simulink model "Stateflow_calculator"  (R2016a)
settings: Solver=FixedStepDiscrete  StartTime=0.0  StopTime=10.0  RelTol=1e-3
settings Model: Creator=Mohamed Fawzy  LastModifiedBy=Mohamed Fawzy
settings OptimizationCC: DefaultParameterBehavior=Inlined  OptimizeModelRefInitCode=on  LifeSpan=1
settings RTWCC: SystemTargetFile=ert.tlc  GenCodeOnly=on  GenerateMakefile=off  TemplateMakefile=ert_default_tmf  GenerateReport=on  IncludeHyperlinkInReport=on  LaunchReport=on  GenerateTraceInfo=on  GenerateTraceReport=on  GenerateTraceReportSl=on  GenerateTraceReportSf=on  GenerateTraceReportEml=on
settings CodeAppCC: ForceParamTrailComments=on  IgnoreCustomStorageClasses=off  OperatorAnnotations=on  SimulinkDataObjDesc=on  SFDataObjDesc=on  MATLABFcnDesc=on  InsertBlockDesc=on  MATLABSourceComments=on
settings ERTTargetCC: GenerateSampleERTMain=on  SuppressErrorStatus=on  InlinedParameterPlacement=NonHierarchical  ERTCustomFileTemplate=example_file_process.tlc

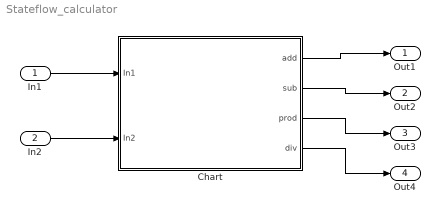
== system Stateflow_calculator ==
  In1 : Inport  OutDataTypeStr=uint8
  In2 : Inport  Port=2  OutDataTypeStr=uint8
  Chart : Stateflow chart  TreatAsAtomicUnit=on
  Out1 : Outport  OutDataTypeStr=uint8
  Out2 : Outport  Port=2  OutDataTypeStr=uint8
  Out3 : Outport  Port=3  OutDataTypeStr=uint16
  Out4 : Outport  Port=4  OutDataTypeStr=uint16
  wires:
  Chart/1(add) -> Out1/1
  Chart/2(sub) -> Out2/1
  Chart/3(prod) -> Out3/1
  Chart/4(div) -> Out4/1
  In1/1 -> Chart/1(In1)
  In2/1 -> Chart/2(In2)

== stateflow chart Stateflow_calculator/Chart ==
  state State
    en:
    add(In1,In2);
    sub(In1,In2);
    product(In1,In2);
    divide(In1,In2);
    du:
    ex:
  state divide(x, y) [function]
    (default) -> (junction 29) : /* zerocheck */
    (junction 29) -> (junction 30) [order 1] : [y==0]
    (junction 29) -> (junction 31) [order 2] : {div = x/y;}
    (junction 30) -> (junction 32) : {div = -1;}
    (junction 32) -> (junction 31)
    (junction 31) -> (junction 33)
  state sub(x,y) [function]
    (default) -> (junction 8) : {sub=(x-y);}
  state product(x,y) [function]
    (default) -> (junction 11) : {prod=(x*y);}
  state add(x,y) [function]
    (default) -> (junction 5) : {add=(x+y);}
  (default) -> State
  data: x function_input uint8; y function_input uint8; x function_input uint8; y function_input uint8; x function_input uint8; y function_input uint8; x function_input uint8; y function_input uint8; In1 input uint8; In2 input uint8; add output uint8; sub output uint8; prod output uint16; div output uint16
